simulink model "PROVA__14_10"  (R2020b)
settings: Solver=FixedStepDiscrete  StartTime=0.0  StopTime=Inf  FixedStep=0.02  RelTol=1e-3  EnableMultiTasking=on
undefined symbols (not defined in the file or in its folder): attuatore_Amax, attuatore_Amin, attuatore_Emax, attuatore_Emin, attuatore_Rmax, attuatore_Rmin, attuatore_Tmax, attuatore_Tmin, DiscIntNeverNeededParam, interventoA_05, interventoA_1, interventoE_05, interventoE_1, interventoT, inv_A, inv_comp_h, inv_E, inv_R, inv_T, K_AW_B_AP_quota, K_AW_B_becc, K_AW_B_imb, K_AW_B_roll, K_imb_inv, Kd_h_app, Kd_h_flare, Ki_AP_quota_select, Ki_AP_rotta, Ki_AP_vel, Ki_becch, Ki_h_app, Ki_h_cruise, Ki_h_flare, Ki_roll, Kp_AP_quota_hold_h, Kp_AP_quota_hold_l, Kp_AP_quota_select, Kp_AP_rotta, Kp_AP_vel, Kp_becch, Kp_comp_h, Kp_h_app_max, Kp_h_app_min, Kp_h_cruise, Kp_h_flare, Kp_imb, Kp_p, Kp_q, Kp_roll, Kp_Rotta_ATO, Newton, phi_max, phi_min, Raphson, safe_phi, safe_V, t_AP, theta_max, theta_min, time_alarm_SAFE ... (+5)
libraries: simulink_extras x34, arduinolib x24, pid_lib x8, simulink x3, dspsigops x3, svdutilitieslib x3, aerolibtransform2sys x2, aerolibtransform2 x2
(part 1 of 7)
Description:
  | Modalita test loop interni
settings Model: SimulationMode=external  ExtModeTrigDuration=2  Creator=luc94  LastModifiedBy=lapis-dspace
settings DataIOCC: ReturnWorkspaceOutputs=off
settings OptimizationCC: EnhancedBackFolding=on  PassReuseOutputArgsAs=Individual arguments  MaxStackSize=64  OptimizeBlockOrder=speed  DifferentSizesBufferReuse=on  OptimizationCustomize=off  EfficientTunableParamExpr=on
settings DebuggingCC: ParameterTunabilityLossMsg=error  ArithmeticOperatorsInVariantConditions=warning
settings HardwareCC: ProdBitPerPointer=32  ProdBitPerSizeT=32  ProdBitPerPtrDiffT=32  ProdLargestAtomicInteger=Long  ProdLargestAtomicFloat=Double  ProdWordSize=32  ProdHWDeviceType=ARM Compatible->ARM Cortex
settings SFSimCC: MATLABDynamicMemAlloc=off  CustomCodeUndefinedFunction=UseInterfaceOnly
settings RTWCC: Description=Embedded Coder  SystemTargetFile=ert.tlc  HardwareBoard=Arduino Due  TemplateMakefile=ert_default_tmf  GenerateReport=on  Toolchain=Arduino ARM  BuildConfiguration=Faster Runs  IncludeHyperlinkInReport=on  LaunchReport=on  GenerateTraceInfo=on  GenerateTraceReport=on  GenerateTraceReportSl=on  GenerateTraceReportSf=on  GenerateTraceReportEml=on
settings CodeAppCC: ForceParamTrailComments=on  IgnoreCustomStorageClasses=off  OperatorAnnotations=on  SimulinkDataObjDesc=on  SFDataObjDesc=on  InsertBlockDesc=on
settings ERTTargetCC: SupportContinuousTime=on  SupportVariableSizeSignals=on

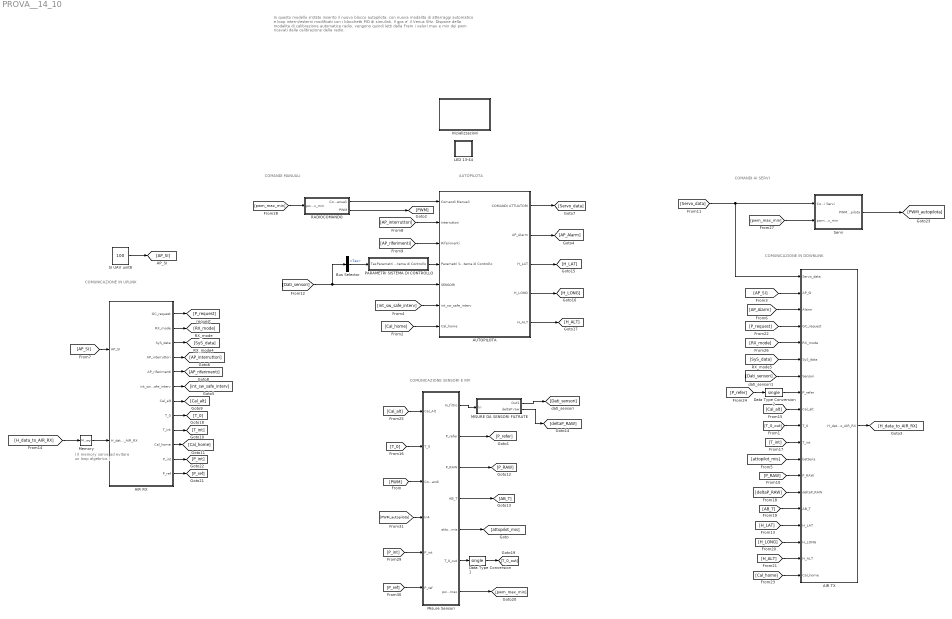
== system PROVA__14_10 ==
  note: In questo modello e'stato inserito il nuovo blocco autopilota, con nuova modalita di atterraggi
      | automatico e loop interni/esterni modificati con i blocchetti PID di simulink.
      | Il gps e' il Venus 5Hz.
      | Dispone della modalita di calibrazione automatica radio, vengono quindi letti dalla Fram i valori max
      | e min dei pwm ricavati dalla calibrazione della radio.
  note: ( Il memory serve ad evitare
      | un loop algebrico.)
  note: COMUNICAZIONE IN UPLINK
  note: COMUNICAZIONE IN DOWNLINK
  note: AUTOPILOTA
  note: COMANDI MANUALI
  note: COMANDI AI SERVI
  note: COMUNICAZIONE SENSORI E RPI
  AIR RX : Subsystem
  AIR TX : Subsystem
  AUTOPILOTA : Subsystem
  Bus Selector : BusSelector  OutputSignals=Tas
  Data Type Conversion1 : DataTypeConversion  OutDataTypeStr=single
  Data Type Conversion2 : DataTypeConversion  OutDataTypeStr=single
  Inizializzazioni : Subsystem
  LED 13-44 : Subsystem
  MISURE DA SENSORI FILTRATE : Subsystem
  Memory : Memory
  Misure Sensori : Subsystem
  PARAMETRI SISTEMA DI CONTROLLO : Subsystem
  RADIOCOMANDO : Subsystem
  SI UAV uint8 : Constant  Value=100  OutDataTypeStr=uint8
  Servi : Subsystem
  wires:
  SI UAV uint8/1 -> [AP_SI]
  AIR RX/4(AP_interruttori) -> [AP_interruttori]
  AIR RX/3(SyS_data) -> [SyS_data]
  AIR RX/6(int_sw_safe_interv) -> [int_sw_safe_interv]
  AIR RX/1(GC_request) -> [P_request]
  AIR RX/5(AP_riferimenti) -> [AP_riferimenti]
  AIR RX/7(Cal_alt) -> [Cal_alt]
  AIR RX/9(T_int) -> [T_int]
  [AP_SI] -> AIR RX/1(AP_SI)
  AIR RX/8(T_0) -> [T_0]
  AIR RX/10(Cal_home) -> [Cal_home]
  [H_data_to_AIR_RX] -> Memory/1
  Memory/1 -> AIR RX/2(H_data_to_AIR_RX)
  AIR RX/2(RX_mode) -> [RX_mode]
  [P_request] -> AIR TX/4(GC_request)
  [Servo_data] -> AIR TX/1(Servo_data), Servi/1(Comandi Servi)
  [Cal_alt] -> AIR TX/9(Cal_alt)
  [RX_mode] -> AIR TX/5(RX_mode)
  [Cal_home] -> AIR TX/19(Cal_home)
  [deltaP_RAW] -> AIR TX/14(deltaP_RAW)
  [attopilot_mis] -> AIR TX/12(batteria)
  [P_refer] -> Data Type Conversion2/1
  [P_RAW] -> AIR TX/13(P_RAW)
  [SyS_data] -> AIR TX/6(SyS_data)
  [H_ALT] -> AIR TX/18(H_ALT)
  Data Type Conversion2/1 -> AIR TX/8(P_refer)
  [H_LAT] -> AIR TX/16(H_LAT)
  [AP_Alarm] -> AIR TX/3(Alarm)
  [T_0_out] -> AIR TX/10(T_0)
  [H_LONG] -> AIR TX/17(H_LONG)
  [AB_T] -> AIR TX/15(AB_T)
  [Dati_sensori] -> AIR TX/7(Sensori)
  [T_int] -> AIR TX/11(T_int)
  AIR TX/1(H_data_to_AIR_RX) -> [H_data_to_AIR_RX]
  [AP_SI] -> AIR TX/2(AP_SI)
  MISURE DA SENSORI FILTRATE/2(deltaP raw) -> [deltaP_RAW]
  Misure Sensori/6(T_0_out) -> Data Type Conversion1/1
  Data Type Conversion1/1 -> [T_0_out]
  Misure Sensori/2(P_refer) -> [P_refer]
  MISURE DA SENSORI FILTRATE/1(Out1) -> [Dati_sensori]
  Misure Sensori/3(P_RAW) -> [P_RAW]
  [Cal_alt] -> Misure Sensori/1(Cal_Alt)
  Misure Sensori/4(AB_T) -> [AB_T]
  Misure Sensori/5(attopilot_mis) -> [attopilot_mis]
  [T_0] -> Misure Sensori/2(T_0)
  Misure Sensori/1(In_filtro) -> MISURE DA SENSORI FILTRATE/1(In)
  [PWM] -> Misure Sensori/3(Comandi)
  Misure Sensori/7(pwm_min_max) -> [pwm_max_min]
  [pwm_max_min] -> Servi/2(pwm_max_min)
  [Cal_home] -> AUTOPILOTA/7(Cal_home)
  AUTOPILOTA/4(H_LONG) -> [H_LONG]
  AUTOPILOTA/5(H_ALT) -> [H_ALT]
  AUTOPILOTA/3(H_LAT) -> [H_LAT]
  [AP_riferimenti] -> AUTOPILOTA/3(Riferimenti)
  RADIOCOMANDO/2(PWM) -> [PWM]
  Bus Selector/1 -> PARAMETRI SISTEMA DI CONTROLLO/1(Tas)  "<Tas>"
  PARAMETRI SISTEMA DI CONTROLLO/1(Parametri Sistema di Controllo) -> AUTOPILOTA/4(Parametri Sistema di Controllo)
  [AP_interruttori] -> AUTOPILOTA/2("Interruttori ")
  RADIOCOMANDO/1(Comandi Manuali) -> AUTOPILOTA/1(Comandi Manuali)
  AUTOPILOTA/1(COMANDI ATTUATORI) -> [Servo_data]
  AUTOPILOTA/2(AP_Alarm) -> [AP_Alarm]
  [int_sw_safe_interv] -> AUTOPILOTA/6(int_sw_safe_interv)
  [pwm_max_min] -> RADIOCOMANDO/1(pwm_max_min)
  [Dati_sensori] -> Bus Selector/1, AUTOPILOTA/5(SENSORI)
  AIR RX/12(P_ref) -> [P_ref]
  AIR RX/11(P_int) -> [P_int]
  [P_int] -> Misure Sensori/5(P_int)
  [P_ref] -> Misure Sensori/6(P_ref)
  Servi/1(PWM_autopilota) -> [PWM_autopilota]
  [PWM_autopilota] -> Misure Sensori/4(In4)

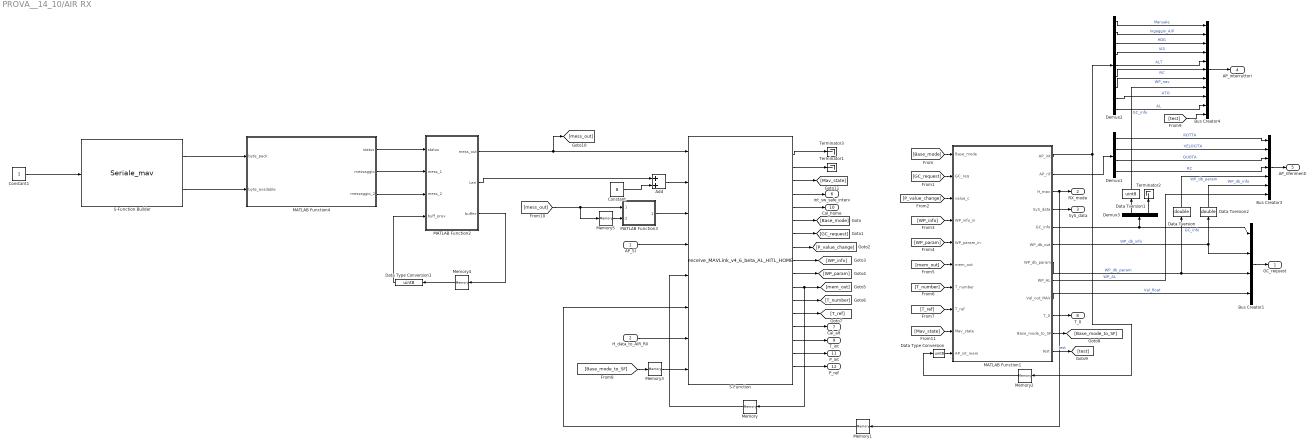
== system PROVA__14_10/AIR RX ==
  AP_SI : Inport
  H_data_to_AIR_RX : Inport  Port=2
  Add : Sum  AccumDataTypeStr=int32
  Bus Creator1 : BusCreator  Inputs=4
  Bus Creator3 : BusCreator  Inputs=7
  Bus Creator4 : BusCreator  Inputs=11
  Constant : Constant  Value=8  OutDataTypeStr=int32  SampleTime=-1
  Constant1 : Constant  OutDataTypeStr=uint8
  Data Tversion : DataTypeConversion  OutDataTypeStr=double
  Data Tversion1 : DataTypeConversion  OutDataTypeStr=uint8
  Data Tversion2 : DataTypeConversion  OutDataTypeStr=double
  Data Type Conversion : DataTypeConversion  OutDataTypeStr=uint8
  Data Type Conversion1 : DataTypeConversion  OutDataTypeStr=uint8
  Demux1 : Demux
  Demux2 : Demux  Outputs=9
  Demux3 : Demux  Outputs=[1 2]
  MATLAB Function1 : MATLAB Function  TreatAsAtomicUnit=on
  MATLAB Function2 : MATLAB Function  TreatAsAtomicUnit=on
  MATLAB Function3 : MATLAB Function  TreatAsAtomicUnit=on
  MATLAB Function4 : MATLAB Function  TreatAsAtomicUnit=on
  Memory : Memory  InheritSampleTime=on
  Memory1 : Memory  InheritSampleTime=on
  Memory2 : Memory  InitialCondition=[0 0 0 0 0 0 0 0 0]
  Memory3 : Memory
  Memory4 : Memory  InitialCondition=uint8(zeros(3,100))  InheritSampleTime=on
  Memory5 : Memory  InheritSampleTime=on
  S-Function : S-Function  FunctionName=receive_MAVLink_v4_6_beta_AL_HITL_HOME  SFunctionModules='receive_MAVLink_v4_6_beta_AL_HITL_HOME_wrapper'  SFunctionDeploymentMode=off  EnableBusSupport=off
  S-Function Builder : S-Function  InitFcn=try, set_param(gcb,'FunctionName','Seriale_mav'), end  FunctionName=Seriale_mav  SFunctionModules=Seriale_mav_wrapper  SFunctionDeploymentMode=off  EnableBusSupport=off  mask(S-Function Builder){}
      mask help: Simulink:masks:SFunctionBuilder_MD
      mask init:
      | val = [[.9  0.75 0.75 1 1 .9 .9 1]',[1 1 0.75 0.75 .9 .9 1 .9]'];try , sys = get_param(gcb,'SfunBuilderFcnName');if isempty(sys), sys = get_param(gcb,'FunctionName'); end,catch, sys = get_param(gcb,'FunctionName'); end
      settings: CopyFcn=set_param(gcbh,'LinkStatus','none')  PreSaveFcn=try, set_param(gcb,'FunctionName','Seriale_mav'), end  OpenFcn=sfunctionwizard(gcbh)
      mask Display: plot(val(:,1),val(:,2)),disp(sys),port_label('input',1,'inutile'),port_label('output',1,'Messaggio'),port_label('output',2,'serial_available')
  Terminator1 : Terminator
  Terminator2 : Terminator
  Terminator3 : Terminator
  GC_request : Outport  VectorParamsAs1DForOutWhenUnconnected=off
  RX_mode : Outport  Port=2  VectorParamsAs1DForOutWhenUnconnected=off
  SyS_data : Outport  Port=3  VectorParamsAs1DForOutWhenUnconnected=off
  AP_interruttori : Outport  Port=4  VectorParamsAs1DForOutWhenUnconnected=off
  AP_riferimenti : Outport  Port=5  VectorParamsAs1DForOutWhenUnconnected=off
  int_sw_safe_interv : Outport  Port=6  VectorParamsAs1DForOutWhenUnconnected=off
  Cal_alt : Outport  Port=7  VectorParamsAs1DForOutWhenUnconnected=off
  T_0 : Outport  Port=8  VectorParamsAs1DForOutWhenUnconnected=off
  T_int : Outport  Port=9  VectorParamsAs1DForOutWhenUnconnected=off
  Cal_home : Outport  Port=10  VectorParamsAs1DForOutWhenUnconnected=off
  P_int : Outport  Port=11  VectorParamsAs1DForOutWhenUnconnected=off
  P_ref : Outport  Port=12  VectorParamsAs1DForOutWhenUnconnected=off
  wires:
  H_data_to_AIR_RX/1 -> S-Function/7
  Memory1/1 -> S-Function/6
  Memory/1 -> S-Function/5
  Memory3/1 -> S-Function/8
  AP_SI/1 -> S-Function/4
  S-Function/5 -> Cal_home/1
  S-Function/4 -> int_sw_safe_interv/1
  S-Function/3 -> [Mav_state]
  S-Function/2 -> Terminator1/1
  S-Function/1 -> Terminator3/1
  S-Function/15 -> T_int/1
  S-Function/14 -> Cal_alt/1
  S-Function/13 -> [T_ref]
  S-Function/12 -> [T_number]
  S-Function/11 -> Memory/1, [mem_out]
  S-Function/10 -> [WP_param]
  S-Function/9 -> [WP_info]
  S-Function/8 -> [P_value_change]
  S-Function/6 -> [Base_mode]
  S-Function/7 -> [GC_request]
  Demux2/6 -> Bus Creator4/6  "RC"
  Data Tversion1/1 -> Bus Creator4/8  "GC_info"
  Memory2/1 -> Data Type Conversion/1
  Bus Creator1/1 -> GC_request/1
  Demux1/2 -> Bus Creator3/2  "VELOCITA"
  Demux2/5 -> Bus Creator4/5  "ALT"
  Demux2/1 -> Bus Creator4/1  "Manuale"
  Demux2/3 -> Bus Creator4/3  "HDG"
  [P_value_change] -> MATLAB Function1/3(value_c)
  Demux1/4 -> Bus Creator3/4  "RC"
  MATLAB Function1/2(AP_rif) -> Demux1/1
  Demux2/8 -> Bus Creator4/9  "ATO"
  MATLAB Function1/7(WP_db_param) -> Bus Creator1/3, Data Tversion/1  "WP_db_param"
  [GC_request] -> MATLAB Function1/2(GC_req)
  Demux2/2 -> Bus Creator4/2  "Ingaggio_A/P"
  [mem_out] -> MATLAB Function1/6(mem_out)
  Bus Creator4/1 -> AP_interruttori/1
  MATLAB Function1/4(SyS_data) -> SyS_data/1
  MATLAB Function1/6(WP_db_out) -> Data Tversion2/1, Bus Creator1/2  "WP_db_info"
  [Mav_state] -> MATLAB Function1/9(Mav_state)
  Demux2/7 -> Bus Creator4/7  "WP_nav"
  [T_ref] -> MATLAB Function1/8(T_ref)
  Data Type Conversion/1 -> MATLAB Function1/10(AP_int_mem)
  Data Tversion2/1 -> Bus Creator3/6  "WP_db_info"
  Demux3/2 -> Terminator2/1
  [Base_mode] -> MATLAB Function1/1(Base_mode)
  [WP_param] -> MATLAB Function1/5(WP_param_in)
  Data Tversion/1 -> Bus Creator3/5  "WP_db_param"
  Demux3/1 -> Data Tversion1/1
  MATLAB Function1/3(H_mav) -> Memory1/1, RX_mode/1
  MATLAB Function1/9(Val_out_MAV) -> Bus Creator1/4  "Val_float"
  Bus Creator3/1 -> AP_riferimenti/1
  [T_number] -> MATLAB Function1/7(T_number)
  MATLAB Function1/5(GC_info) -> Demux3/1, Bus Creator1/1  "GC_info"
  MATLAB Function1/1(AP_int) -> Demux2/1, Memory2/1
  [WP_info] -> MATLAB Function1/4(WP_info_in)
  [Base_mode_to_SF] -> Memory3/1
  MATLAB Function1/11(Base_mode_to_SF) -> [Base_mode_to_SF]
  Demux1/3 -> Bus Creator3/3  "QUOTA"
  MATLAB Function1/12(test) -> [test]  "test"
  Demux2/4 -> Bus Creator4/4  "IAS"
  [test] -> Bus Creator4/11
  Demux1/1 -> Bus Creator3/1  "ROTTA"
  MATLAB Function1/8(WP_AL) -> Bus Creator3/7  "WP_AL"
  MATLAB Function1/10(T_0) -> T_0/1
  Demux2/9 -> Bus Creator4/10  "AL"
  MATLAB Function4/3(messaggio_2) -> MATLAB Function2/3(mess_2)
  MATLAB Function2/2(Len) -> Add/1
  MATLAB Function4/1(status) -> MATLAB Function2/1(status)
  MATLAB Function4/2(messaggio) -> MATLAB Function2/2(mess_1)
  Memory4/1 -> Data Type Conversion1/1
  MATLAB Function2/3(buffer) -> Memory4/1
  Constant/1 -> Add/2
  MATLAB Function2/1(mess_out) -> S-Function/1, [mess_out]
  MATLAB Function3/1(new_mex) -> S-Function/3
  Add/1 -> S-Function/2
  Data Type Conversion1/1 -> MATLAB Function2/4(buff_prev)
  Memory5/1 -> MATLAB Function3/2(mess_out_prev)
  [mess_out] -> Memory5/1, MATLAB Function3/1(mess_out)
  S-Function Builder/2 -> MATLAB Function4/2(byte_available)
  S-Function Builder/1 -> MATLAB Function4/1(byte_pack)
  Constant1/1 -> S-Function Builder/1
  S-Function/16 -> P_int/1
  S-Function/17 -> P_ref/1

== system PROVA__14_10/AIR TX ==
  Servo_data : Inport
  AP_SI : Inport  Port=2
  Alarm : Inport  Port=3
  GC_request : Inport  Port=4
  RX_mode : Inport  Port=5
  SyS_data : Inport  Port=6
  Sensori : Inport  Port=7
  P_refer : Inport  Port=8
  Cal_alt : Inport  Port=9
  T_0 : Inport  Port=10
  T_int : Inport  Port=11
  batteria : Inport  Port=12
  P_RAW : Inport  Port=13
  deltaP_RAW : Inport  Port=14
  AB_T : Inport  Port=15
  H_LAT : Inport  Port=16
  H_LONG : Inport  Port=17
  H_ALT : Inport  Port=18
  Cal_home : Inport  Port=19
  Data Type Conversion : DataTypeConversion  OutDataTypeStr=single
  Data Type Conversion1 : DataTypeConversion  OutDataTypeStr=single
  Data Type Conversion2 : DataTypeConversion  OutDataTypeStr=int16
  "Enable " : Subsystem  TreatAsAtomicUnit=on
  GPS : Subsystem  SystemSampleTime=0.02
  Ground : Ground
  Heartbeat : Subsystem  SystemSampleTime=1
  IMU & Attidude : Subsystem  SystemSampleTime=0.04
  If_subsystem : Subsystem
  Memory : Memory
  Pa to hPa : Gain  Gain=0.01
  Pa to hPa1 : Gain  Gain=0.01
  S-Function : S-Function  FunctionName=send_MAVLink_v4_4_2_beta_3_HOME  SFunctionModules='send_MAVLink_v4_4_2_beta_3_HOME_wrapper'  SFunctionDeploymentMode=off  EnableBusSupport=off
  Servo : Subsystem  SystemSampleTime=0.5
  SystemStatus : Subsystem  SystemSampleTime=0.2
  VFR : Subsystem  SystemSampleTime=0.5
  Waypoints : Subsystem  SystemSampleTime=1
  H_data_to_AIR_RX : Outport  VectorParamsAs1DForOutWhenUnconnected=off
  wires:
  If_subsystem/2(time) -> S-Function/2
  If_subsystem/1(iflogic) -> S-Function/1
  VFR/2(Heading) -> S-Function/20
  Heartbeat/2(H_data) -> H_data_to_AIR_RX/1, S-Function/13
  Alarm/1 -> SystemStatus/2(Alarm), Heartbeat/1(Alarm)
  RX_mode/1 -> Heartbeat/2(RX_mode)
  S-Function/1 -> "Enable "/Enable
  T_0/1 -> S-Function/26
  AP_SI/1 -> S-Function/3
  deltaP_RAW/1 -> Pa to hPa1/1
  Sensori/1 -> GPS/1(GPS1), IMU & Attidude/1(AHRS1), Waypoints/2("Sensori "), Servo/1(Sensor), VFR/1(VFR1)
  SyS_data/1 -> SystemStatus/1(SyS_input)
  S-Function/3 -> "Enable "/2(In2)
  SystemStatus/1(onboard) -> S-Function/8
  SystemStatus/4(B_remaining) -> S-Function/11
  T_int/1 -> S-Function/27
  SystemStatus/2(LVDE) -> S-Function/9
  Heartbeat/1(custom) -> S-Function/12
  Cal_alt/1 -> S-Function/25
  GC_request/1 -> Waypoints/1(GC_req)
  S-Function/4 -> Memory/1
  S-Function/2 -> "Enable "/1(In1)
  GPS/3(hdg1) -> S-Function/18
  Waypoints/2(P_value) -> S-Function/5
  IMU & Attidude/2(ATT) -> S-Function/15
  Servo_data/1 -> Servo/2(Servo)
  Memory/1 -> S-Function/23
  Data Type Conversion1/1 -> S-Function/29
  Waypoints/1(GC_info) -> S-Function/4
  Servo/1(Servo_data) -> S-Function/22
  GPS/2(vel) -> S-Function/17
  IMU & Attidude/1(IMU) -> S-Function/14
  AB_T/1 -> Data Type Conversion2/1
  Pa to hPa/1 -> Data Type Conversion/1
  P_RAW/1 -> Pa to hPa/1
  Waypoints/3(WP_info) -> S-Function/6
  Pa to hPa1/1 -> Data Type Conversion1/1
  batteria/1 -> SystemStatus/3(batteria)
  P_refer/1 -> S-Function/24
  Data Type Conversion/1 -> S-Function/28
  GPS/1(LLAA) -> S-Function/16
  Data Type Conversion2/1 -> S-Function/30
  H_ALT/1 -> S-Function/34
  SystemStatus/3(B_current) -> S-Function/10
  Cal_home/1 -> S-Function/31
  VFR/3(Throttle) -> S-Function/21
  Waypoints/4(WP_param) -> S-Function/7
  H_LAT/1 -> S-Function/32
  VFR/1(AGAC) -> S-Function/19
  H_LONG/1 -> S-Function/33
  Ground/1 -> S-Function/35

== system PROVA__14_10/AUTOPILOTA ==
  note: SISTEMA DI GESTIONE
  note: LOOP ESTERNI e SWITCH
  note: LOOP INTERNI e SWITCH
  note: MODI A/P
  Comandi Manuali : Inport
  "Interruttori " : Inport  Port=2
  Riferimenti : Inport  Port=3
  Parametri Sistema di Controllo : Inport  Port=4
  SENSORI : Inport  Port=5
  int_sw_safe_interv : Inport  Port=6
  Cal_home : Inport  Port=7
  AUTOPILOTI1 : Subsystem
  CONTROLLI INTERNI E SWITCH1 : Subsystem
  Demux : Demux  Outputs=2
  GESTIONE AUTOPILOTI1 : Subsystem
  Mux : Mux  Inputs=2
  Subsystem1 : Subsystem
  Terminator : Terminator
  COMANDI ATTUATORI : Outport  VectorParamsAs1DForOutWhenUnconnected=off
  AP_Alarm : Outport  Port=2  VectorParamsAs1DForOutWhenUnconnected=off
  H_LAT : Outport  Port=3  VectorParamsAs1DForOutWhenUnconnected=off
  H_LONG : Outport  Port=4  VectorParamsAs1DForOutWhenUnconnected=off
  H_ALT : Outport  Port=5  VectorParamsAs1DForOutWhenUnconnected=off
  wires:
  Comandi Manuali/1 -> AUTOPILOTI1/6(comandi), CONTROLLI INTERNI E SWITCH1/2(Comandi Manuali), GESTIONE AUTOPILOTI1/3(Comandi Manuali)
  CONTROLLI INTERNI E SWITCH1/1(Comandi Attuatori) -> COMANDI ATTUATORI/1
  GESTIONE AUTOPILOTI1/1(Switch Attuatori) -> Subsystem1/6(Switch_attuatori), AUTOPILOTI1/7(Switch attuatori), CONTROLLI INTERNI E SWITCH1/4(Switch Attuatori)
  Parametri Sistema di Controllo/1 -> AUTOPILOTI1/2(Parametri Sistema di Controllo), CONTROLLI INTERNI E SWITCH1/1(Parametri Sistema di Controllo)
  GESTIONE AUTOPILOTI1/6(Switch_ATO) -> [Switch_ATO]
  Subsystem1/4(Riferimenti) -> AUTOPILOTI1/3(Riferimenti)
  Demux/2 -> GESTIONE AUTOPILOTI1/5(int_sw_intervento)
  GESTIONE AUTOPILOTI1/7(Switch_AL) -> [Switch_AL]
  [Switch_AL] -> CONTROLLI INTERNI E SWITCH1/7(Switch_AL)
  AUTOPILOTI1/1(Riferimento Manetta) -> CONTROLLI INTERNI E SWITCH1/3(Riferimento Manetta)
  [Switch_ATO] -> CONTROLLI INTERNI E SWITCH1/6(Switch_ATO)
  [Switch_AL] -> AUTOPILOTI1/9(Switch_AL)
  GESTIONE AUTOPILOTI1/4(Alarm Intervento) -> Mux/2
  "Interruttori "/1 -> GESTIONE AUTOPILOTI1/2("Interruttori "), Subsystem1/2(Interruttori)
  [Switch_ATO] -> AUTOPILOTI1/8(Switch_ATO)
  Cal_home/1 -> Subsystem1/5(Cal_home)
  Mux/1 -> AP_Alarm/1
  Demux/1 -> GESTIONE AUTOPILOTI1/4(int_sw_safe)
  int_sw_safe_interv/1 -> Demux/1
  Subsystem1/1(H_LAT) -> H_LAT/1
  GESTIONE AUTOPILOTI1/5(Alarm Safe) -> AUTOPILOTI1/5(Alarm Safe), Mux/1
  Subsystem1/3(H_ALT) -> H_ALT/1
  GESTIONE AUTOPILOTI1/3(modo) -> Subsystem1/4(modo)
  Subsystem1/2(H_LONG) -> H_LONG/1
  SENSORI/1 -> GESTIONE AUTOPILOTI1/1(Sensori), Subsystem1/1(sensori), AUTOPILOTI1/1(Sensori), CONTROLLI INTERNI E SWITCH1/5(Sensori)
  GESTIONE AUTOPILOTI1/2(Riferimenti Safe) -> AUTOPILOTI1/4(Riferimenti Safe)
  Riferimenti/1 -> Subsystem1/3(waypoints e riferimenti vettoriali)
  Subsystem1/5(Inner_loop_ATO) -> CONTROLLI INTERNI E SWITCH1/8(Inner_loop_ATO)
  CONTROLLI INTERNI E SWITCH1/2(theta_track) -> AUTOPILOTI1/10(traking theta)
  CONTROLLI INTERNI E SWITCH1/3(manetta_track) -> AUTOPILOTI1/11(manetta_track)
  AUTOPILOTI1/2(Riferimenti Rollio e Beccheggio) -> Terminator/1
  CONTROLLI INTERNI E SWITCH1/4(phi_track) -> AUTOPILOTI1/12(track_phi)

== system PROVA__14_10/Inizializzazioni ==
  S-Function Builder : S-Function  FunctionName=Risoluzione_12bit  SFunctionModules=Risoluzione_12bit_wrapper  SFunctionDeploymentMode=off  EnableBusSupport=off  mask(S-Function Builder){}
      mask help: Simulink:masks:SFunctionBuilder_MD
      mask init: same as PROVA__14_10/AIR RX/S-Function Builder
      settings: CopyFcn=set_param(gcbh,'LinkStatus','none')  PreSaveFcn=try, set_param(gcb,'FunctionName','Risoluzione_12bit'), end  OpenFcn=sfunctionwizard(gcbh)
      mask Display:
      | plot(val(:,1),val(:,2))
      | disp(sys)

== system PROVA__14_10/LED 13-44 ==
  Digital Output : arduinolib/Digital Output  pinNumber=13  Direction=output  blockPlatform=arduino
  Digital Output1 : arduinolib/Digital Output  pinNumber=44  Direction=output  blockPlatform=arduino
  Pulse Generator : DiscretePulseGenerator  Period=25  PulseWidth=2  SampleTime=0.04
  Pulse Generator1 : DiscretePulseGenerator  Period=25  PulseWidth=2  SampleTime=0.04
  wires:
  Pulse Generator/1 -> Digital Output/1
  Pulse Generator1/1 -> Digital Output1/1

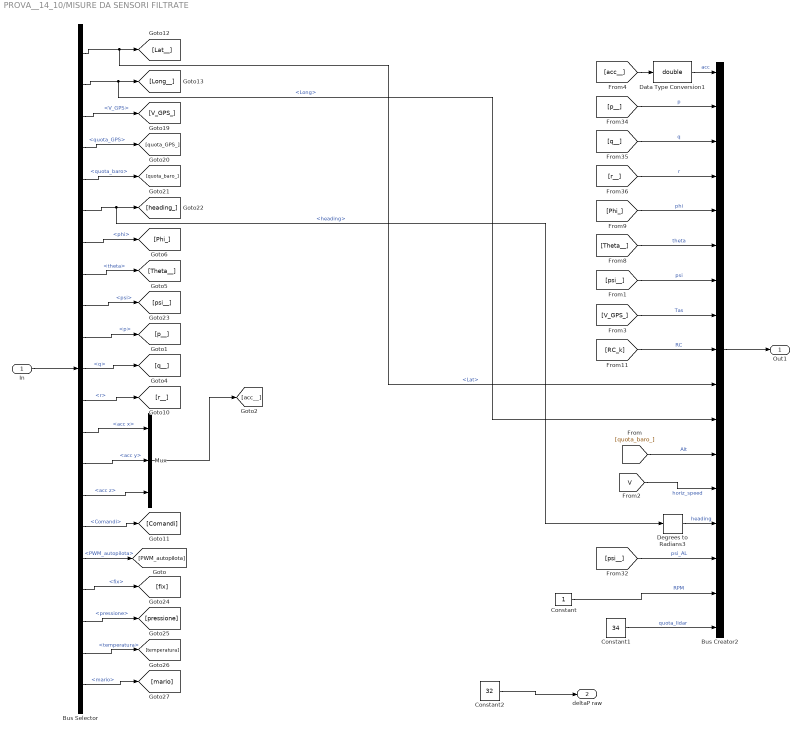
== system PROVA__14_10/MISURE DA SENSORI FILTRATE ==
  In : Inport
  Bus Creator2 : BusCreator  Inputs=17
  Bus Selector : BusSelector  OutputSignals=Lat,Long,V_GPS,quota_GPS,quota_baro,heading,phi,theta,psi,p,q,r,acc x,acc y,acc z,Comandi,PWM_autopilota,fix,pressione,temperatura,mario
  Constant : Constant  OutDataTypeStr=double  SampleTime=0.02
  Constant1 : Constant  Value=34
  Constant2 : Constant  Value=32
  Data Type Conversion1 : DataTypeConversion  OutDataTypeStr=double
  Degrees to Radians3 : simulink_extras/Transformations/Degrees to Radians
  Mux : Mux  Inputs=3
  Out1 : Outport  VectorParamsAs1DForOutWhenUnconnected=off
  deltaP raw : Outport  Port=2
  wires:
  In/1 -> Bus Selector/1
  Bus Selector/4 -> [quota_GPS_]  "<quota_GPS>"
  Bus Selector/9 -> [psi__]  "<psi>"
  Bus Selector/10 -> [p__]  "<p>"
  Bus Selector/11 -> [q__]  "<q>"
  Bus Selector/12 -> [r__]  "<r>"
  Bus Selector/7 -> [Phi_]  "<phi>"
  Bus Selector/8 -> [Theta__]  "<theta>"
  Bus Selector/13 -> Mux/1  "<acc x>"
  Bus Selector/14 -> Mux/2  "<acc y>"
  Bus Selector/15 -> Mux/3  "<acc z>"
  Mux/1 -> [acc__]
  Bus Selector/16 -> [Comandi]  "<Comandi>"
  [psi__] -> Bus Creator2/7  "psi"
  [Phi_] -> Bus Creator2/5  "phi"
  Bus Selector/1 -> Bus Creator2/10, [Lat__]  "<Lat>"
  [RC_k] -> Bus Creator2/9  "RC"
  [q__] -> Bus Creator2/3  "q"
  [p__] -> Bus Creator2/2  "p"
  Bus Selector/6 -> Degrees to Radians3/1, [heading_]  "<heading>"
  Constant/1 -> Bus Creator2/16  "RPM"
  [Theta__] -> Bus Creator2/6  "theta"
  Bus Selector/3 -> [V_GPS_]  "<V_GPS>"
  Bus Selector/2 -> Bus Creator2/11, [Long__]  "<Long>"
  [V_GPS_] -> Bus Creator2/8  "Tas"
  [r__] -> Bus Creator2/4  "r"
  [acc__] -> Data Type Conversion1/1
  Bus Selector/5 -> [quota_baro_]  "<quota_baro>"
  Bus Creator2/1 -> Out1/1
  Data Type Conversion1/1 -> Bus Creator2/1  "acc"
  [psi__] -> Bus Creator2/15  "psi_AL"
  Bus Selector/18 -> [fix]  "<fix>"
  Bus Selector/19 -> [pressione]  "<pressione>"
  Bus Selector/20 -> [temperatura]  "<temperatura>"
  Bus Selector/21 -> [mario]  "<mario>"
  Constant1/1 -> Bus Creator2/17  "quota_lidar"
  Degrees to Radians3/1 -> Bus Creator2/14  "heading"
  Bus Selector/17 -> [PWM_autopilota]  "<PWM_autopilota>"
  [quota_baro_] -> Bus Creator2/12  "Alt"
  [V] -> Bus Creator2/13  "horiz_speed"
  Constant2/1 -> deltaP raw/1

== system PROVA__14_10/Misure Sensori ==
  Cal_Alt : Inport
  T_0 : Inport  Port=2
  Comandi : Inport  Port=3
  In4 : Inport  Port=4
  P_int : Inport  Port=5
  P_ref : Inport  Port=6
  ATTOPILOT : Subsystem  Commented=on
  BMP_280 : Subsystem
  Bus Creator : BusCreator  Inputs=21
  Constant : Constant  Value=[0 0 0]
  Data Type Conversion1 : DataTypeConversion  OutDataTypeStr=double
  Demux : Demux  Outputs=6
  Demux1 : Demux  Outputs=9
  GPS_Venus : Subsystem
  MTi : Subsystem
  In_filtro : Outport  VectorParamsAs1DForOutWhenUnconnected=off
  P_refer : Outport  Port=2  VectorParamsAs1DForOutWhenUnconnected=off
  P_RAW : Outport  Port=3  VectorParamsAs1DForOutWhenUnconnected=off
  AB_T : Outport  Port=4  VectorParamsAs1DForOutWhenUnconnected=off
  attopilot_mis : Outport  Port=5  VectorParamsAs1DForOutWhenUnconnected=off
  T_0_out : Outport  Port=6  VectorParamsAs1DForOutWhenUnconnected=off
  pwm_min_max : Outport  Port=7  VectorParamsAs1DForOutWhenUnconnected=off
  wires:
  Demux/3 -> Bus Creator/3  "V_GPS"
  T_0/1 -> BMP_280/2(T_0)
  Constant/1 -> attopilot_mis/1
  Cal_Alt/1 -> BMP_280/1(Cal_Alt), GPS_Venus/1(Cal_alt)
  Demux/4 -> Bus Creator/4  "quota_GPS"
  Demux1/5 -> Bus Creator/12  "q"
  Demux1/9 -> Bus Creator/16  "psi"
  Demux1/7 -> Bus Creator/14  "phi"
  Demux1/2 -> Bus Creator/9  "acc y"
  Demux1/3 -> Bus Creator/10  "acc z"
  Demux1/6 -> Bus Creator/13  "r"
  Demux1/1 -> Bus Creator/8  "acc x"
  Demux/2 -> Bus Creator/2  "Long"
  Demux1/8 -> Bus Creator/15  "theta"
  Demux1/4 -> Bus Creator/11  "p"
  Bus Creator/1 -> In_filtro/1
  Demux/1 -> Bus Creator/1  "Lat"
  Demux/5 -> Bus Creator/5  "heading"
  Data Type Conversion1/1 -> Demux1/1
  GPS_Venus/1(Misure_GPS) -> Demux/1
  MTi/1(Misure MTi) -> Data Type Conversion1/1
  BMP_280/2(P_refer) -> P_refer/1
  BMP_280/3(P_RAW) -> P_RAW/1, Bus Creator/18  "pressione"
  BMP_280/4(AB_T) -> AB_T/1, Bus Creator/19  "temperatura"
  BMP_280/5(T_0_out) -> T_0_out/1
  BMP_280/1(h_) -> Bus Creator/17  "quota_baro"
  Comandi/1 -> Bus Creator/7  "Comandi"
  BMP_280/6("pwm_max_min ") -> pwm_min_max/1
  Demux/6 -> Bus Creator/6  "fix"
  GPS_Venus/2(mario) -> [mario]
  [mario] -> Bus Creator/20  "mario"
  P_int/1 -> BMP_280/3(P_int)
  P_ref/1 -> BMP_280/4(P_ref)
  In4/1 -> Bus Creator/21  "PWM_autopilota"

== system PROVA__14_10/PARAMETRI SISTEMA DI CONTROLLO ==
  Tas : Inport
  Bus Creator1 : BusCreator  Inputs=19
  Gain3 : Gain  Gain=-1
  K AntiWindup-Bumpless AP quota : Constant  Value=K_AW_B_AP_quota  OutDataTypeStr=int16
  K AntiWindup-Bumpless controllore beccheggio : Constant  Value=K_AW_B_becc  OutDataTypeStr=single
  K AntiWindup-Bumpless controllore imbardata : Constant  Value=K_AW_B_imb  OutDataTypeStr=int8
  K AntiWindup-Bumpless controllore rollio : Constant  Value=K_AW_B_roll  OutDataTypeStr=int16
  K AntiWindup-Bumpless controllore rollio1 : Constant  Commented=on  Value=500  OutDataTypeStr=int16
  K controllo imbardata inversa : Constant  Value=K_imb_inv  OutDataTypeStr=int8
  Ki AP quota Select : Constant  Value=Ki_AP_quota_select  OutDataTypeStr=single
  Ki AP rotta1 : Constant  Value=Ki_AP_rotta  OutDataTypeStr=single
  Ki AP velocità : Constant  Value=Ki_AP_vel  OutDataTypeStr=single
  Ki controllore  beccheggio1 : Constant  Value=Ki_becch  OutDataTypeStr=single
  Ki controllore  rollio1 : Constant  Commented=on  Value=0.013  OutDataTypeStr=single
  Ki controllore  rollio2 : Constant  Commented=on  Value=0.025  OutDataTypeStr=single
  Ki controllore  rollio3 : Constant  Value=Ki_roll  OutDataTypeStr=single
  Kp AP quota Hold2 : Constant  Commented=on  Value=0.15  OutDataTypeStr=single
  Kp AP quota Select : Constant  Value=Kp_AP_quota_select  OutDataTypeStr=single
  Kp AP rotta : Constant  Value=Kp_AP_rotta  OutDataTypeStr=single
  Kp AP rotta1 : Constant  Commented=on  Value=0.3  OutDataTypeStr=single
  Kp AP velocità : Constant  Value=Kp_AP_vel  OutDataTypeStr=single
  Kp controllore  rollio1 : Constant  Commented=on  Value=0.15  OutDataTypeStr=single
  Kp controllore  rollio2 : Constant  Commented=on  Value=0.13  OutDataTypeStr=single
  Kp controllore  rollio3 : Constant  Value=Kp_roll  OutDataTypeStr=single
  Kp controllore  velocità rollio1 : Constant  Commented=on  Value=0.04  OutDataTypeStr=single
  Kp controllore  velocità rollio2 : Constant  Commented=on  Value=0.05  OutDataTypeStr=single
  Kp controllore  velocità rollio3 : Constant  Value=Kp_p  OutDataTypeStr=single
  Kp controllore beccheggio1 : Constant  Value=Kp_becch  OutDataTypeStr=single
  Kp controllore imbardata : Constant  Value=Kp_imb  OutDataTypeStr=single
  Kp controllore imbardata1 : Constant  Commented=on  Value=-0.1  OutDataTypeStr=single
  Kp controllore velocità beccheggio1 : Constant  Value=Kp_q  OutDataTypeStr=single
  Saturation : Saturate  UpperLimit=Kp_AP_quota_hold_l  LowerLimit=Kp_AP_quota_hold_h
  n-D Lookup Table : Lookup_n-D  NumberOfTableDimensions=1  BreakpointsForDimension1=[V_stall V_max*0.8]  Table=[Kp_AP_quota_hold_l Kp_AP_quota_hold_h]  RndMeth=Simplest  InputSameDT=on
  Parametri Sistema di Controllo : Outport  VectorParamsAs1DForOutWhenUnconnected=off
  wires:
  Gain3/1 -> Bus Creator1/19  "K_imb_inv"
  Bus Creator1/1 -> Parametri Sistema di Controllo/1  "Cond.Volo.Richiesta"
  Kp controllore imbardata/1 -> Bus Creator1/7  "Kp_imb"
  Kp AP velocità/1 -> Bus Creator1/8  "Kp_AP_vel"
  Saturation/1 -> Bus Creator1/10  "Kp_AP_quota_hold"
  Kp AP quota Select/1 -> Bus Creator1/11  "Kp_AP_quota_select"
  Ki AP quota Select/1 -> Bus Creator1/12  "Ki_AP_quota_select"
  Kp AP rotta/1 -> Bus Creator1/13  "Kp_AP_rotta"
  K AntiWindup-Bumpless controllore beccheggio/1 -> Bus Creator1/15  "K_AW-B_becc"
  K AntiWindup-Bumpless controllore rollio/1 -> Bus Creator1/16  "K_AW-B_roll"
  K AntiWindup-Bumpless controllore imbardata/1 -> Bus Creator1/17  "K_AW-B_imb"
  K AntiWindup-Bumpless AP quota/1 -> Bus Creator1/18  "K_AW-B_AP_quota"
  Ki AP velocità/1 -> Bus Creator1/9  "Ki_AP_vel"
  Ki AP rotta1/1 -> Bus Creator1/14  "Ki_AP_rotta"
  Kp controllore  rollio3/1 -> Bus Creator1/4  "Kp_roll"
  Kp controllore  velocità rollio3/1 -> Bus Creator1/6  "Kp_p"
  Ki controllore  rollio3/1 -> Bus Creator1/5  "Ki_roll"
  n-D Lookup Table/1 -> Saturation/1
  Tas/1 -> n-D Lookup Table/1
  Kp controllore beccheggio1/1 -> Bus Creator1/1  "Kp_becch"
  Ki controllore  beccheggio1/1 -> Bus Creator1/2  "Ki_becch"
  Kp controllore velocità beccheggio1/1 -> Bus Creator1/3  "Kp_q"
  K controllo imbardata inversa/1 -> Gain3/1  "K_imb_inv"

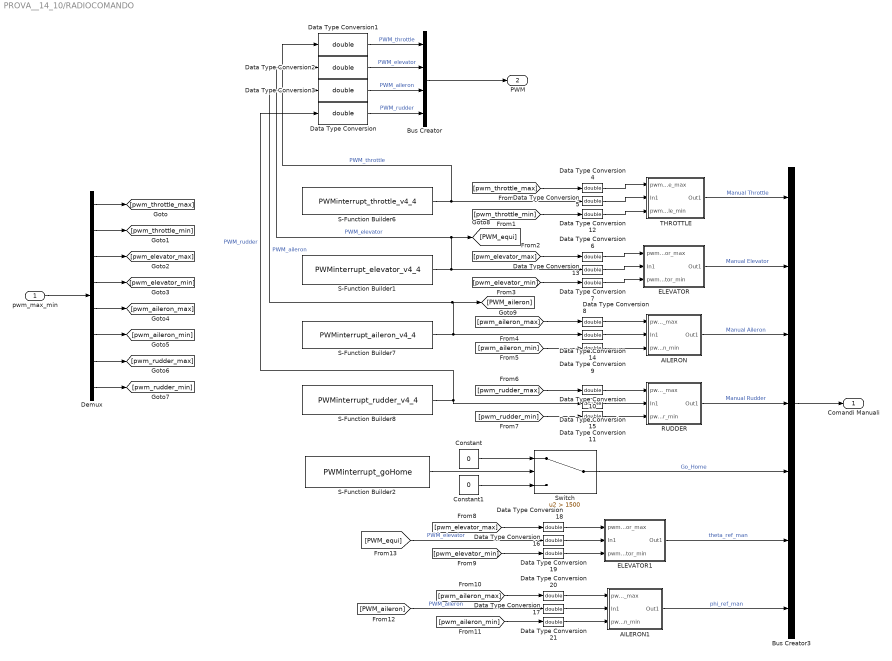
== system PROVA__14_10/RADIOCOMANDO ==
  pwm_max_min : Inport
  AILERON : Subsystem
  AILERON1 : Subsystem
  Bus Creator : BusCreator  Inputs=4
  Bus Creator3 : BusCreator  Inputs=7
  Constant : Constant  Value=0
  Constant1 : Constant  Value=0
  Data Type Conversion{,1..21} (22 alike) : DataTypeConversion  OutDataTypeStr=double
  Demux : Demux  Outputs=8
  ELEVATOR : Subsystem
  ELEVATOR1 : Subsystem
  RUDDER : Subsystem
  S-Function Builder1 : S-Function  InitFcn=try, set_param(gcb,'FunctionName','PWMinterrupt_elevator_v4_4'), end  FunctionName=PWMinterrupt_elevator_v4_4  SFunctionModules=PWMinterrupt_elevator_v4_4_wrapper calcInputElevator  SFunctionDeploymentMode=off  EnableBusSupport=off  mask(S-Function Builder){}
      mask init: same as PROVA__14_10/AIR RX/S-Function Builder
      settings: CopyFcn=set_param(gcbh,'LinkStatus','none')  PreSaveFcn=try, set_param(gcb,'FunctionName','PWMinterrupt_elevator_v4_4'), end  OpenFcn=sfunctionwizard(gcbh)
      mask Display: plot(val(:,1),val(:,2)),disp(sys), port_label('output',1,'out')
  S-Function Builder2 : S-Function  InitFcn=try, set_param(gcb,'FunctionName','PWMinterrupt_goHome'), end  FunctionName=PWMinterrupt_goHome  SFunctionModules=PWMinterrupt_goHome_wrapper calcInput_go_Home  SFunctionDeploymentMode=off  EnableBusSupport=off  mask(S-Function Builder){}
      mask init: same as PROVA__14_10/AIR RX/S-Function Builder
      settings: CopyFcn=set_param(gcbh,'LinkStatus','none')  PreSaveFcn=try, set_param(gcb,'FunctionName','PWMinterrupt_goHome'), end  OpenFcn=sfunctionwizard(gcbh)
      mask Display: plot(val(:,1),val(:,2)),disp(sys), port_label('output',1,'out')
  S-Function Builder6 : S-Function  InitFcn=try, set_param(gcb,'FunctionName','PWMinterrupt_throttle_v4_4'), end  FunctionName=PWMinterrupt_throttle_v4_4  SFunctionModules=PWMinterrupt_throttle_v4_4_wrapper calcInputThrottle  SFunctionDeploymentMode=off  EnableBusSupport=off  mask(S-Function Builder){}
      mask init: same as PROVA__14_10/AIR RX/S-Function Builder
      settings: CopyFcn=set_param(gcbh,'LinkStatus','none')  PreSaveFcn=try, set_param(gcb,'FunctionName','PWMinterrupt_throttle_v4_4'), end  OpenFcn=sfunctionwizard(gcbh)
      mask Display: plot(val(:,1),val(:,2)),disp(sys),port_label('output',1,'out')
  S-Function Builder7 : S-Function  InitFcn=try, set_param(gcb,'FunctionName','PWMinterrupt_aileron_v4_4'), end  FunctionName=PWMinterrupt_aileron_v4_4  SFunctionModules=PWMinterrupt_aileron_v4_4_wrapper calcInputAileron  SFunctionDeploymentMode=off  EnableBusSupport=off  mask(S-Function Builder){}
      mask init: same as PROVA__14_10/AIR RX/S-Function Builder
      settings: CopyFcn=set_param(gcbh,'LinkStatus','none')  PreSaveFcn=try, set_param(gcb,'FunctionName','PWMinterrupt_aileron_v4_4'), end  OpenFcn=sfunctionwizard(gcbh)
      mask Display: plot(val(:,1),val(:,2)),disp(sys), port_label('output',1,'out')
  S-Function Builder8 : S-Function  InitFcn=try, set_param(gcb,'FunctionName','PWMinterrupt_rudder_v4_4'), end  FunctionName=PWMinterrupt_rudder_v4_4  SFunctionModules=PWMinterrupt_rudder_v4_4_wrapper calcInputRudder  SFunctionDeploymentMode=off  EnableBusSupport=off  mask(S-Function Builder){}
      mask init: same as PROVA__14_10/AIR RX/S-Function Builder
      settings: CopyFcn=set_param(gcbh,'LinkStatus','none')  PreSaveFcn=try, set_param(gcb,'FunctionName','PWMinterrupt_rudder_v4_4'), end  OpenFcn=sfunctionwizard(gcbh)
      mask Display: plot(val(:,1),val(:,2)),disp(sys),port_label('output',1,'out')
  Switch : Switch  Criteria=u2 > Threshold  Threshold=1500
  THROTTLE : Subsystem
  Comandi Manuali : Outport  VectorParamsAs1DForOutWhenUnconnected=off
  PWM : Outport  Port=2  VectorParamsAs1DForOutWhenUnconnected=off
  wires:
  Bus Creator3/1 -> Comandi Manuali/1
  S-Function Builder2/1 -> Switch/2
  Constant/1 -> Switch/1
  Constant1/1 -> Switch/3
  Switch/1 -> Bus Creator3/5  "Go_Home"
  S-Function Builder8/1 -> Data Type Conversion15/1, Data Type Conversion/1  "PWM_rudder"
  S-Function Builder1/1 -> Data Type Conversion2/1, [PWM_equi], Data Type Conversion13/1  "PWM_elevator"
  S-Function Builder7/1 -> [PWM_aileron], Data Type Conversion3/1, Data Type Conversion14/1  "PWM_aileron"
  S-Function Builder6/1 -> Data Type Conversion1/1, Data Type Conversion5/1  "PWM_throttle"
  THROTTLE/1(Out1) -> Bus Creator3/1  "Manual Throttle"
  ELEVATOR/1(Out1) -> Bus Creator3/2  "Manual Elevator"
  AILERON/1(Out1) -> Bus Creator3/3  "Manual Aileron"
  RUDDER/1(Out1) -> Bus Creator3/4  "Manual Rudder"
  Bus Creator/1 -> PWM/1
  Data Type Conversion1/1 -> Bus Creator/1  "PWM_throttle"
  Data Type Conversion2/1 -> Bus Creator/2  "PWM_elevator"
  Data Type Conversion3/1 -> Bus Creator/3  "PWM_aileron"
  Data Type Conversion/1 -> Bus Creator/4  "PWM_rudder"
  pwm_max_min/1 -> Demux/1
  Demux/1 -> [pwm_throttle_max]
  Demux/2 -> [pwm_throttle_min]
  Demux/3 -> [pwm_elevator_max]
  Demux/4 -> [pwm_elevator_min]
  Demux/5 -> [pwm_aileron_max]
  Demux/6 -> [pwm_aileron_min]
  Demux/8 -> [pwm_rudder_min]
  Demux/7 -> [pwm_rudder_max]
  [pwm_elevator_min] -> Data Type Conversion7/1
  [pwm_elevator_max] -> Data Type Conversion6/1
  [pwm_aileron_min] -> Data Type Conversion9/1
  [pwm_aileron_max] -> Data Type Conversion8/1
  [pwm_rudder_max] -> Data Type Conversion10/1
  [pwm_rudder_min] -> Data Type Conversion11/1
  [pwm_throttle_max] -> Data Type Conversion4/1
  [pwm_throttle_min] -> Data Type Conversion12/1
  Data Type Conversion6/1 -> ELEVATOR/1(pwm_elevator_max)
  Data Type Conversion7/1 -> ELEVATOR/3(pwm_elevator_min)
  Data Type Conversion8/1 -> AILERON/1(pwm_aileron_max)
  Data Type Conversion9/1 -> AILERON/3(pwm_aileron_min)
  Data Type Conversion10/1 -> RUDDER/1(pwm_rudder_max)
  Data Type Conversion11/1 -> RUDDER/3(pwm_rudder_min)
  Data Type Conversion4/1 -> THROTTLE/1(pwm_throttle_max)
  Data Type Conversion5/1 -> THROTTLE/2(In1)
  Data Type Conversion12/1 -> THROTTLE/3(pwm_throttle_min)
  Data Type Conversion13/1 -> ELEVATOR/2(In1)
  Data Type Conversion14/1 -> AILERON/2(In1)
  Data Type Conversion15/1 -> RUDDER/2(In1)
  [pwm_aileron_max] -> Data Type Conversion20/1
  AILERON1/1(Out1) -> Bus Creator3/7  "phi_ref_man"
  [PWM_equi] -> Data Type Conversion16/1  "PWM_elevator"
  ELEVATOR1/1(Out1) -> Bus Creator3/6  "theta_ref_man"
  [pwm_elevator_min] -> Data Type Conversion19/1
  Data Type Conversion17/1 -> AILERON1/2(In1)
  [pwm_aileron_min] -> Data Type Conversion21/1
  Data Type Conversion21/1 -> AILERON1/3(pwm_aileron_min)
  Data Type Conversion18/1 -> ELEVATOR1/1(pwm_elevator_max)
  Data Type Conversion16/1 -> ELEVATOR1/2(In1)
  Data Type Conversion20/1 -> AILERON1/1(pwm_aileron_max)
  Data Type Conversion19/1 -> ELEVATOR1/3(pwm_elevator_min)
  [pwm_elevator_max] -> Data Type Conversion18/1
  [PWM_aileron] -> Data Type Conversion17/1  "PWM_aileron"

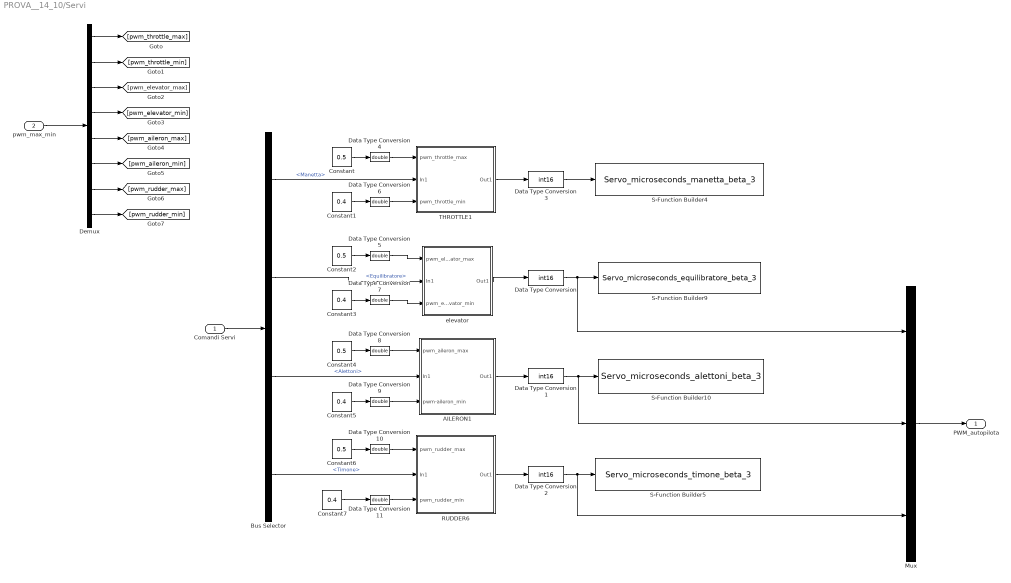
== system PROVA__14_10/Servi ==
  Comandi Servi : Inport
  pwm_max_min : Inport  Port=2
  AILERON1 : Subsystem
  Bus Selector : BusSelector  OutputSignals=Manetta,Equilibratore,Alettoni,Timone
  Constant{,2,4,6} (4 alike) : Constant  Value=0.5
  Constant{1,3,5,7} (4 alike) : Constant  Value=0.4
  Data Type Conversion{,1..3} (4 alike) : DataTypeConversion  OutDataTypeStr=int16
  Data Type Conversion{4..11} (8 alike) : DataTypeConversion  OutDataTypeStr=double
  Demux : Demux  Outputs=8
  Mux : Mux  Inputs=3
  RUDDER6 : Subsystem
  S-Function Builder10 : S-Function  InitFcn=try, set_param(gcb,'FunctionName','Servo_microseconds_alettoni_beta_3'), end  FunctionName=Servo_microseconds_alettoni_beta_3  SFunctionModules=Servo_microseconds_alettoni_beta_3_wrapper Servo  SFunctionDeploymentMode=off  EnableBusSupport=off  mask(S-Function Builder){}
      mask help: Simulink:masks:SFunctionBuilder_MD
      mask init: same as PROVA__14_10/AIR RX/S-Function Builder
      settings: CopyFcn=set_param(gcbh,'LinkStatus','none')  PreSaveFcn=try, set_param(gcb,'FunctionName','Servo_microseconds_alettoni_beta_3'), end  OpenFcn=sfunctionwizard(gcbh)
      mask DialogControl DescTextVar Prompt: Send PWM to servo using servo.wirtemicrosecond() function. Select Pin from which sends the PWM signal.
      mask Display: plot(val(:,1),val(:,2)),disp(sys),port_label('input',1,'tau')
  S-Function Builder4 : S-Function  InitFcn=try, set_param(gcb,'FunctionName','Servo_microseconds_manetta_beta_3'), end  FunctionName=Servo_microseconds_manetta_beta_3  SFunctionModules=Servo_microseconds_manetta_beta_3_wrapper Servo  SFunctionDeploymentMode=off  EnableBusSupport=off  mask(S-Function Builder){}
      mask help: Simulink:masks:SFunctionBuilder_MD
      mask init: same as PROVA__14_10/AIR RX/S-Function Builder
      settings: CopyFcn=set_param(gcbh,'LinkStatus','none')  PreSaveFcn=try, set_param(gcb,'FunctionName','Servo_microseconds_manetta_beta_3'), end  OpenFcn=sfunctionwizard(gcbh)
      mask DialogControl DescTextVar Prompt: Send PWM to servo using servo.wirtemicrosecond() function. Select Pin from which sends the PWM signal.
      mask Display: plot(val(:,1),val(:,2)),disp(sys),port_label('input',1,'tau')
  S-Function Builder5 : S-Function  InitFcn=try, set_param(gcb,'FunctionName','Servo_microseconds_timone_beta_3'), end  FunctionName=Servo_microseconds_timone_beta_3  SFunctionModules=Servo_microseconds_timone_beta_3_wrapper Servo  SFunctionDeploymentMode=off  EnableBusSupport=off  mask(S-Function Builder){}
      mask help: Simulink:masks:SFunctionBuilder_MD
      mask init: same as PROVA__14_10/AIR RX/S-Function Builder
      settings: CopyFcn=set_param(gcbh,'LinkStatus','none')  PreSaveFcn=try, set_param(gcb,'FunctionName','Servo_microseconds_timone_beta_3'), end  OpenFcn=sfunctionwizard(gcbh)
      mask DialogControl DescTextVar Prompt: Send PWM to servo using servo.wirtemicrosecond() function. Select Pin from which sends the PWM signal.
      mask Display: plot(val(:,1),val(:,2)),disp(sys), port_label('input',1,'tau')
  S-Function Builder9 : S-Function  InitFcn=try, set_param(gcb,'FunctionName','Servo_microseconds_equilibratore_beta_3'), end  FunctionName=Servo_microseconds_equilibratore_beta_3  SFunctionModules=Servo_microseconds_equilibratore_beta_3_wrapper Servo  SFunctionDeploymentMode=off  EnableBusSupport=off  mask(S-Function Builder){}
      mask help: Simulink:masks:SFunctionBuilder_MD
      mask init: same as PROVA__14_10/AIR RX/S-Function Builder
      settings: CopyFcn=set_param(gcbh,'LinkStatus','none')  PreSaveFcn=try, set_param(gcb,'FunctionName','Servo_microseconds_equilibratore_beta_3'), end  OpenFcn=sfunctionwizard(gcbh)
      mask DialogControl DescTextVar Prompt: Send PWM to servo using servo.wirtemicrosecond() function. Select Pin from which sends the PWM signal.
      mask Display: plot(val(:,1),val(:,2)),disp(sys),port_label('input',1,'tau')
  THROTTLE1 : Subsystem
  elevator : Subsystem
  PWM_autopilota : Outport  VectorParamsAs1DForOutWhenUnconnected=off
  wires:
  AILERON1/1(Out1) -> Data Type Conversion1/1
  THROTTLE1/1(Out1) -> Data Type Conversion3/1
  RUDDER6/1(Out1) -> Data Type Conversion2/1
  elevator/1(Out1) -> Data Type Conversion/1
  Bus Selector/1 -> THROTTLE1/2(In1)  "<Manetta>"
  Bus Selector/4 -> RUDDER6/2(In1)  "<Timone>"
  Bus Selector/3 -> AILERON1/2(In1)  "<Alettoni>"
  Bus Selector/2 -> elevator/2(In1)  "<Equilibratore>"
  Comandi Servi/1 -> Bus Selector/1
  Demux/3 -> [pwm_elevator_max]
  Demux/2 -> [pwm_throttle_min]
  Demux/6 -> [pwm_aileron_min]
  Demux/1 -> [pwm_throttle_max]
  pwm_max_min/1 -> Demux/1
  Demux/8 -> [pwm_rudder_min]
  Demux/7 -> [pwm_rudder_max]
  Demux/5 -> [pwm_aileron_max]
  Demux/4 -> [pwm_elevator_min]
  Constant/1 -> Data Type Conversion4/1
  Constant1/1 -> Data Type Conversion6/1
  Constant2/1 -> Data Type Conversion5/1
  Constant3/1 -> Data Type Conversion7/1
  Constant4/1 -> Data Type Conversion8/1
  Constant5/1 -> Data Type Conversion9/1
  Constant6/1 -> Data Type Conversion10/1
  Constant7/1 -> Data Type Conversion11/1
  Data Type Conversion/1 -> Mux/1, S-Function Builder9/1
  Data Type Conversion1/1 -> Mux/2, S-Function Builder10/1
  Data Type Conversion3/1 -> S-Function Builder4/1
  Data Type Conversion2/1 -> Mux/3, S-Function Builder5/1
  Data Type Conversion4/1 -> THROTTLE1/1(pwm_throttle_max)
  Data Type Conversion6/1 -> THROTTLE1/3(pwm_throttle_min)
  Data Type Conversion5/1 -> elevator/1(pwm_elevator_max)
  Data Type Conversion7/1 -> elevator/3(pwm_elevator_min)
  Data Type Conversion8/1 -> AILERON1/1(pwm_aileron_max)
  Data Type Conversion9/1 -> AILERON1/3(pwm-aileron_min)
  Data Type Conversion10/1 -> RUDDER6/1(pwm_rudder_max)
  Data Type Conversion11/1 -> RUDDER6/3("pwm_rudder_min ")
  Mux/1 -> PWM_autopilota/1

== system PROVA__14_10/AIR TX/Enable  ==
  In1 : Inport
  In2 : Inport  Port=2
  Enable : EnablePort
  Chart : Stateflow chart  TreatAsAtomicUnit=on
  wires:
  In2/1 -> Chart/2(Len)
  In1/1 -> Chart/1(datain)

== system PROVA__14_10/AIR TX/GPS ==
  note: NB.: se non si posside un dato inserire una costante con valore 0. I dati vanno messi tutti anche se zeri nell'ordine elencato
  note: Vanno inseriti i collegamenti con i dati provenienti dal sensore GPS
      | in uscita bisogna dare 3 segnali:
      |
      | -LLAA: latitudine, longitudine, altitudine, altitudine relativa
      | -VEL: velocità (x,y,z)
      | -HDG: heading
  GPS1 : Inport
  Bus Selector : BusSelector  OutputSignals=Lat,Long,Alt,horiz_speed,RC,heading
  Data Type Conversion : DataTypeConversion  OutDataTypeStr=int32  RndMeth=Simplest
  Data Type Conversion1 : DataTypeConversion  OutDataTypeStr=int16  RndMeth=Simplest
  Data Type Conversion2 : DataTypeConversion  OutDataTypeStr=uint16  RndMeth=Simplest
  Gain : Gain  Gain=[10^7;10^7;1000 ;1000]
  Gain1 : Gain  Gain=100
  Gain2 : Gain  Gain=100
  Mux : Mux
  Mux1 : Mux  Inputs=3
  Radians to Degrees : simulink_extras/Transformations/Radians to Degrees
  Radians to Degrees1 : simulink_extras/Transformations/Radians to Degrees
  alt_r : Constant  Value=0
  vel y : Constant  Value=0  OutDataTypeStr=double
  LLAA : Outport  VectorParamsAs1DForOutWhenUnconnected=off
  vel : Outport  Port=2  VectorParamsAs1DForOutWhenUnconnected=off
  hdg1 : Outport  Port=3  VectorParamsAs1DForOutWhenUnconnected=off
  wires:
  Radians to Degrees1/1 -> Mux/2
  Radians to Degrees/1 -> Mux/1
  Gain2/1 -> Data Type Conversion2/1
  Gain/1 -> Data Type Conversion/1
  Gain1/1 -> Data Type Conversion1/1
  Mux/1 -> Gain/1
  Bus Selector/6 -> Gain2/1  "<heading>"
  Bus Selector/5 -> Mux1/3  "<RC>"
  Mux1/1 -> Gain1/1  "VEL"
  alt_r/1 -> Mux/4
  GPS1/1 -> Bus Selector/1
  Bus Selector/1 -> Radians to Degrees/1  "<Lat>"
  Bus Selector/2 -> Radians to Degrees1/1  "<Long>"
  Bus Selector/3 -> Mux/3  "<Alt>"
  Bus Selector/4 -> Mux1/1  "<horiz_speed>"
  vel y/1 -> Mux1/2
  Data Type Conversion2/1 -> hdg1/1
  Data Type Conversion1/1 -> vel/1
  Data Type Conversion/1 -> LLAA/1

== system PROVA__14_10/AIR TX/Heartbeat ==
  note: Vanno inseriti i collegamenti con i dati provenienti dalla ricezione (stazione di terra) e gli allarmi
      | in uscita bisogna dare 2 vettori costituiti da:
      | -I:
      | -custom code (su può mettere ciò che si vuole)
      | -II:
      | -vettore di 2 componenti: tido di veivolo e tipo di autopilota
      | -vettore di due componenti che è creato tramite la matlabfuncition
  Alarm : Inport
  RX_mode : Inport  Port=2
  Alarm set : MATLAB Function  TreatAsAtomicUnit=on
  Constant : Constant  Value=0
  Data Type Conversion : DataTypeConversion  OutDataTypeStr=uint32
  Data Type Conversion1 : DataTypeConversion  OutDataTypeStr=uint8
  Mux : Mux  Inputs=2
  Type fixed_wing Autopilot generic : Constant  Value=[1;0]  OutDataTypeStr=uint8
  custom : Outport  VectorParamsAs1DForOutWhenUnconnected=off
  H_data : Outport  Port=2  VectorParamsAs1DForOutWhenUnconnected=off
  wires:
  Constant/1 -> Data Type Conversion/1
  Data Type Conversion1/1 -> H_data/1
  Data Type Conversion/1 -> custom/1
  RX_mode/1 -> Alarm set/2(Rx_mode)
  Alarm/1 -> Alarm set/1(Alarm)
  Type fixed_wing Autopilot generic/1 -> Mux/1
  Alarm set/1(H_mav) -> Mux/2
  Mux/1 -> Data Type Conversion1/1

== system PROVA__14_10/AIR TX/IMU & Attidude ==
  note: NB.: se non si posside un dato inserire una costante con valore 0. I dati vanno messi tutti anche se zeri nell'ordine elencato
  note: Vanno inseriti i collegamenti con i dati provenienti dal sensore inerziale (MTi)
      | in uscita bisogna dare un vettore di 12 componenti contente in ordine:
      | - 3 accelerazioni (x,y,z)
      | - 3 giroscopiche (p,q,r)
      | - 3 comp. campo magnetico
      | -3 angoli di eulero
  AHRS1 : Inport
  Bus Selector : BusSelector  OutputSignals=acc,p,q,r,phi,theta,psi
  Constant : Constant  Value=0  OutDataTypeStr=double  SampleTime=t_AP
  Constant1 : Constant  Value=0  OutDataTypeStr=double  SampleTime=t_AP
  Constant2 : Constant  Value=0  OutDataTypeStr=double  SampleTime=t_AP
  Data Type Conversion : DataTypeConversion  OutDataTypeStr=int16  RndMeth=Simplest
  Data Type Conversion1 : DataTypeConversion  OutDataTypeStr=single
  Gain : Gain  Gain=10^3
  Mux{1,3..5} (4 alike) : Mux  Inputs=3
  Mux2 : Mux  Inputs=2
  IMU : Outport  VectorParamsAs1DForOutWhenUnconnected=off
  ATT : Outport  Port=2  VectorParamsAs1DForOutWhenUnconnected=off
  wires:
  Constant/1 -> Mux5/1
  Mux4/1 -> Mux2/1
  Bus Selector/7 -> Mux4/3  "<psi>"
  Bus Selector/6 -> Mux4/2  "<theta>"
  Bus Selector/5 -> Mux4/1  "<phi>"
  Mux3/1 -> Mux2/2, Mux1/2
  Bus Selector/4 -> Mux3/3  "<r>"
  Bus Selector/3 -> Mux3/2  "<q>"
  Bus Selector/2 -> Mux3/1  "<p>"
  Bus Selector/1 -> Mux1/1  "<acc>"
  AHRS1/1 -> Bus Selector/1
  Mux2/1 -> Data Type Conversion1/1
  Gain/1 -> Data Type Conversion/1
  Data Type Conversion1/1 -> ATT/1
  Data Type Conversion/1 -> IMU/1
  Mux1/1 -> Gain/1
  Constant1/1 -> Mux5/2
  Mux5/1 -> Mux1/3
  Constant2/1 -> Mux5/3

== system PROVA__14_10/AIR TX/If_subsystem ==
  note: Blocco per la temporizzazione dell'invio dei messaggi
  Data Type Conversion3 : DataTypeConversion  OutDataTypeStr=uint32  RndMeth=Simplest
  Gain : Gain  Gain=100
  Subsystem : Subsystem
  iflogic_function : MATLAB Function  TreatAsAtomicUnit=on
  iflogic : Outport  VectorParamsAs1DForOutWhenUnconnected=off
  time : Outport  Port=2  VectorParamsAs1DForOutWhenUnconnected=off
  wires:
  Subsystem/3(time) -> Gain/1
  Subsystem/2(H_10) -> iflogic_function/2(H10)
  Subsystem/1(H_50) -> iflogic_function/1(H50)
  Gain/1 -> Data Type Conversion3/1
  Data Type Conversion3/1 -> time/1
  iflogic_function/1(iflogic) -> iflogic/1

== system PROVA__14_10/AIR TX/Servo ==
  note: NB.: se non si posside un dato inserire una costante con valore 0. I dati vanno messi tutti anche se zeri nell'ordine elencato
  note: Vanno inseriti i collegamenti con i dati provenienti dal sensore di velocità
      | in uscita bisogna dare 1 segnale composto da:
      |
      | -  PORT
      | -8 servo
  note: La quota lidar la invio come componente 8 dei servi
  Sensor : Inport
  Servo : Inport  Port=2
  Bus Selector : BusSelector  OutputSignals=Manetta,Equilibratore,Alettoni,Timone
  Bus Selector1 : BusSelector  OutputSignals=quota_lidar
  Constant : Constant  Value=4
  Constant1 : Constant  Value=zeros(3,1)
  Conversione : Subsystem
  Data Type Conversion1 : DataTypeConversion  OutDataTypeStr=uint16  RndMeth=Simplest
  Gain : Gain  Gain=100
  Mux : Mux  Inputs=7
  Saturation : Saturate  UpperLimit=4000  LowerLimit=0
  Servo_data : Outport  VectorParamsAs1DForOutWhenUnconnected=off
  wires:
  Conversione/4(Out4) -> Mux/5
  Conversione/3(Out3) -> Mux/4
  Conversione/2(Out2) -> Mux/3
  Conversione/1(Out1) -> Mux/2
  Bus Selector/1 -> Conversione/1(Manetta)  "<Manetta>"
  Bus Selector/4 -> Conversione/4(Timone)  "<Timone>"
  Bus Selector/3 -> Conversione/3(Alettoni)  "<Alettoni>"
  Bus Selector/2 -> Conversione/2(Equilibratore)  "<Equilibratore>"
  Constant1/1 -> Mux/6
  Constant/1 -> Mux/1
  Servo/1 -> Bus Selector/1
  Mux/1 -> Data Type Conversion1/1
  Data Type Conversion1/1 -> Servo_data/1  "Heading"
  Sensor/1 -> Bus Selector1/1
  Bus Selector1/1 -> Gain/1  "<quota_lidar>"
  Gain/1 -> Saturation/1
  Saturation/1 -> Mux/7
